simulink model "Dqo_model_Group_05"  (R2023a)
settings: Solver=VariableStepAuto  StartTime=0.0  StopTime=10.0  RelTol=1e-3
InitFcn:
  | Rs=0.03957
  | Rr=0.02215
  | Ls=0.000389+0.01664 %Lls+Lm
  | Lm=0.01664
  | Lr=0.000389+0.01664 % Llr+Lm
  | J=1.3
  | P=4
  | w=2*pi*60
  | Tl=200.106
settings Model: Creator=shivam  LastModifiedBy=shivam

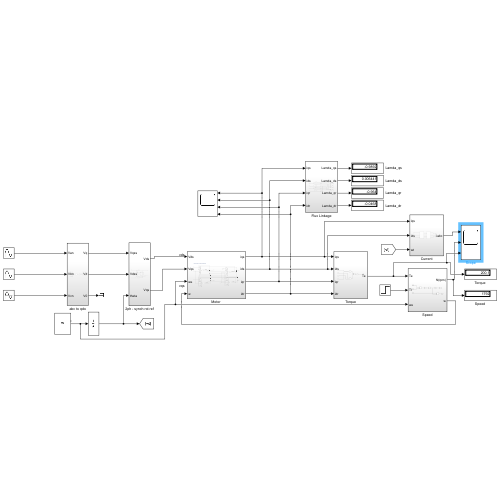
[thumbnail: Simulink's stored preview of the top-level diagram]
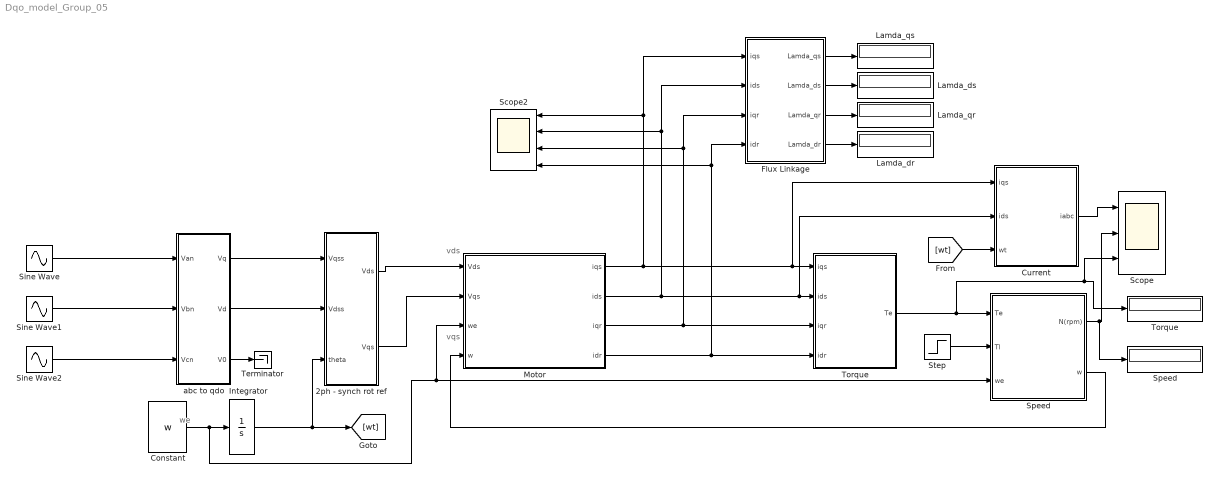
== system Dqo_model_Group_05 ==
  note: we
  note: vqs
  note: vds
  2ph - synch rot ref : Subsystem
  Constant : Constant  Value=w
  Current : Subsystem
  Flux Linkage : Subsystem
  Integrator : Integrator
  Lamda_dr : Display
  Lamda_ds : Display
  Lamda_qr : Display
  Lamda_qs : Display
  "Motor " : Subsystem
  Scope : Scope  NumInputPorts=3
  Scope2 : Scope  NumInputPorts=4
  Sine Wave : Sin  Amplitude=(460*sqrt(2))/sqrt(3)  Frequency=2*pi*60  SampleTime=0
  Sine Wave1 : Sin  Amplitude=(460*sqrt(2))/sqrt(3)  Frequency=2*pi*60  Phase=-(2*pi)/3  SampleTime=0
  Sine Wave2 : Sin  Amplitude=(460*sqrt(2))/sqrt(3)  Frequency=2*pi*60  Phase=(2*pi)/3  SampleTime=0
  Speed : Subsystem
  "Speed " : Display
  Step : Step  After=200.106  SampleTime=0
  Terminator : Terminator
  Torque : Subsystem
  "Torque " : Display
  abc to qdo : Subsystem
  wires:
  "Motor "/3(iqr) -> Torque/3(iqr), Scope2/3, Flux Linkage/3(iqr)
  abc to qdo/3(V0) -> Terminator/1
  2ph - synch rot ref/1(Vds) -> "Motor "/1("Vds ")
  Flux Linkage/4(Lamda_dr) -> Lamda_dr/1
  Speed/1(N(rpm)) -> "Speed "/1, Scope/2
  Constant/1 -> Speed/3(we), "Motor "/3(we), Integrator/1
  abc to qdo/1(Vq) -> 2ph - synch rot ref/1(Vqss)
  Speed/2(w) -> "Motor "/4(w)
  Torque/1("Te ") -> "Torque "/1, Scope/3, Speed/1(Te)
  Integrator/1 -> [wt], 2ph - synch rot ref/3(theta)
  Flux Linkage/1(Lamda_qs) -> Lamda_qs/1
  [wt] -> Current/3(wt)
  Step/1 -> Speed/2(Tl)
  Flux Linkage/2(Lamda_ds) -> Lamda_ds/1
  Sine Wave2/1 -> abc to qdo/3(Vcn)
  Sine Wave1/1 -> abc to qdo/2(Vbn)
  Current/1(iabc) -> Scope/1
  Flux Linkage/3(Lamda_qr) -> Lamda_qr/1
  "Motor "/4(idr) -> Torque/4(idr), Scope2/4, Flux Linkage/4(idr)
  2ph - synch rot ref/2(Vqs) -> "Motor "/2("Vqs ")
  Sine Wave/1 -> abc to qdo/1(Van)
  abc to qdo/2(Vd) -> 2ph - synch rot ref/2(Vdss)
  "Motor "/1(iqs) -> Current/1(iqs), Torque/1(iqs), Flux Linkage/1(iqs), Scope2/1
  "Motor "/2(ids) -> Current/2(ids), Torque/2(ids), Scope2/2, Flux Linkage/2(ids)

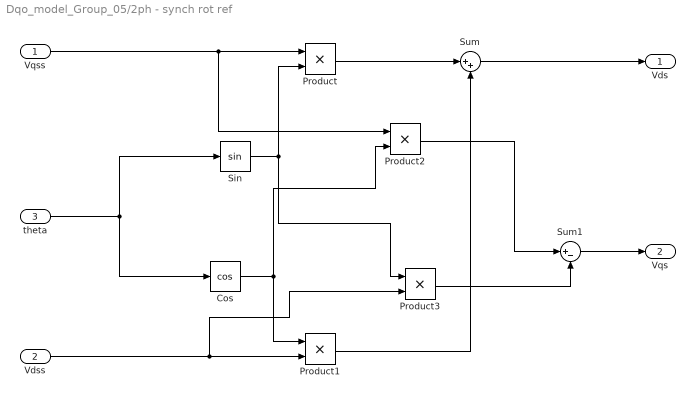
== system Dqo_model_Group_05/2ph - synch rot ref ==
  Vqss : Inport
  Vdss : Inport  Port=2
  theta : Inport  Port=3
  Cos : Trigonometry  Operator=cos
  Product{,1..3} (4 alike) : Product
  Sin : Trigonometry
  Sum : Sum  Inputs=|++
  Sum1 : Sum  Inputs=|+-
  Vds : Outport
  Vqs : Outport  Port=2
  wires:
  theta/1 -> Sin/1, Cos/1
  Vqss/1 -> Product2/1, Product/1
  Sin/1 -> Product/2, Product3/1
  Vdss/1 -> Product3/2, Product1/2
  Cos/1 -> Product1/1, Product2/2
  Product/1 -> Sum/1
  Product1/1 -> Sum/2
  Sum/1 -> Vds/1
  Product2/1 -> Sum1/1
  Product3/1 -> Sum1/2
  Sum1/1 -> Vqs/1

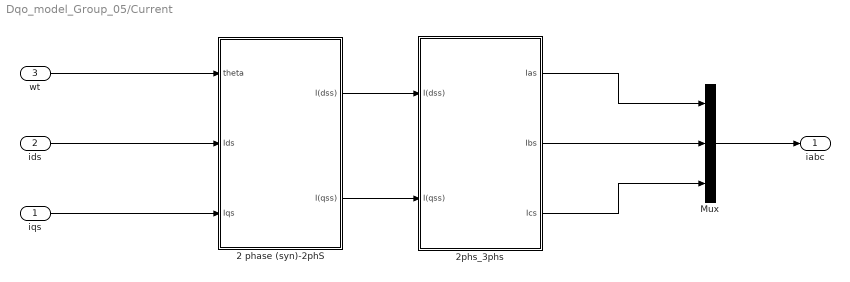
== system Dqo_model_Group_05/Current ==
  iqs : Inport
  ids : Inport  Port=2
  wt : Inport  Port=3
  2 phase (syn)-2phS : Subsystem
  2phs_3phs : Subsystem
  Mux : Mux  Inputs=3
  iabc : Outport  VectorParamsAs1DForOutWhenUnconnected=off
  wires:
  ids/1 -> 2 phase (syn)-2phS/2(Ids)
  iqs/1 -> 2 phase (syn)-2phS/3(Iqs)
  wt/1 -> 2 phase (syn)-2phS/1(theta)
  Mux/1 -> iabc/1
  2 phase (syn)-2phS/1(I(dss)) -> 2phs_3phs/1(I(dss))
  2 phase (syn)-2phS/2(I(qss)) -> 2phs_3phs/2(I(qss))
  2phs_3phs/1(Ias) -> Mux/1
  2phs_3phs/2(Ibs) -> Mux/2
  2phs_3phs/3(Ics) -> Mux/3

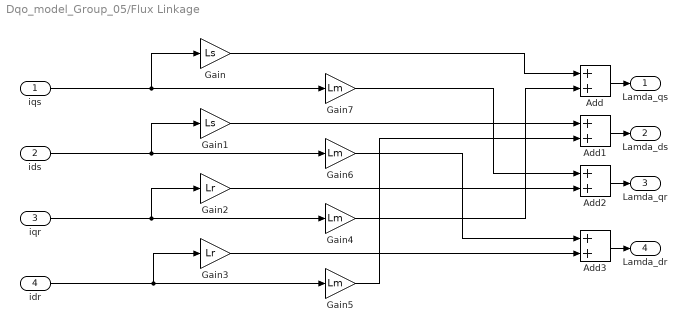
== system Dqo_model_Group_05/Flux Linkage ==
  iqs : Inport
  ids : Inport  Port=2
  iqr : Inport  Port=3
  idr : Inport  Port=4
  Add{,1..3} (4 alike) : Sum
  Gain : Gain  Gain=Ls
  Gain1 : Gain  Gain=Ls
  Gain2 : Gain  Gain=Lr
  Gain3 : Gain  Gain=Lr
  Gain{4..7} (4 alike) : Gain  Gain=Lm
  Lamda_qs : Outport
  Lamda_ds : Outport  Port=2
  Lamda_qr : Outport  Port=3
  Lamda_dr : Outport  Port=4
  wires:
  Gain4/1 -> Add/2
  Gain1/1 -> Add1/1
  ids/1 -> Gain6/1, Gain1/1
  iqs/1 -> Gain7/1, Gain/1
  Gain6/1 -> Add3/1
  idr/1 -> Gain5/1, Gain3/1
  iqr/1 -> Gain4/1, Gain2/1
  Gain5/1 -> Add1/2
  Gain/1 -> Add/1
  Gain7/1 -> Add2/1
  Gain3/1 -> Add3/2
  Add2/1 -> Lamda_qr/1
  Gain2/1 -> Add2/2
  Add/1 -> Lamda_qs/1
  Add3/1 -> Lamda_dr/1
  Add1/1 -> Lamda_ds/1

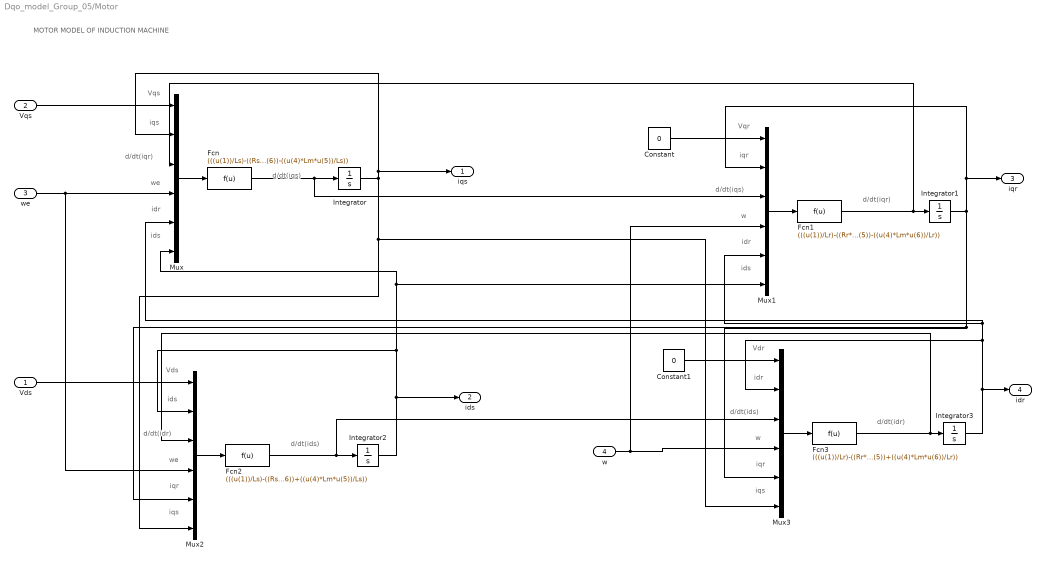
== system Dqo_model_Group_05/Motor  ==
  note: d/dt(iqs)
  note: ids
  note: idr
  note: we
  note: d/dt(iqr)
  note: iqs
  note: Vqs
  note: MOTOR MODEL OF INDUCTION MACHINE
  note: d/dt(iqr)
  note: ids
  note: d/dt(iqs)
  note: w
  note: idr
  note: Vqr
  note: iqr
  note: d/dt(ids)
  note: iqs
  note: d/dt(idr)
  note: we
  note: iqr
  note: Vds
  note: ids
  note: iqr
  note: w
  note: Vdr
  note: d/dt(ids)
  note: idr
  note: iqs
  note: d/dt(idr)
  "Vds " : Inport
  "Vqs " : Inport  Port=2
  we : Inport  Port=3
  w : Inport  Port=4
  Constant : Constant  Value=0
  Constant1 : Constant  Value=0
  Fcn : Fcn  Expr=(((u(1))/Ls)-((Rs*u(2))/Ls)-((u(3)*Lm)/Ls)-(u(4)*u(6))-((u(4)*Lm*u(5))/Ls))
  Fcn1 : Fcn  Expr=(((u(1))/Lr)-((Rr*u(2))/Lr)-((u(3)*Lm)/Lr)-(u(4)*u(5))-((u(4)*Lm*u(6))/Lr))
  Fcn2 : Fcn  Expr=(((u(1))/Ls)-((Rs*u(2))/Ls)-((u(3)*Lm)/Ls)+(u(4)*u(6))+((u(4)*Lm*u(5))/Ls))
  Fcn3 : Fcn  Expr=(((u(1))/Lr)-((Rr*u(2))/Lr)-((u(3)*Lm)/Lr)+(u(4)*u(5))+((u(4)*Lm*u(6))/Lr))
  Integrator{,1..3} (4 alike) : Integrator
  Mux{,1..3} (4 alike) : Mux  Inputs=6
  iqs : Outport  VectorParamsAs1DForOutWhenUnconnected=off
  ids : Outport  Port=2  VectorParamsAs1DForOutWhenUnconnected=off
  iqr : Outport  Port=3  VectorParamsAs1DForOutWhenUnconnected=off
  idr : Outport  Port=4  VectorParamsAs1DForOutWhenUnconnected=off
  wires:
  Integrator3/1 -> idr/1, Mux3/2, Mux1/5, Mux/5
  Mux/1 -> Fcn/1
  Fcn2/1 -> Mux3/3, Integrator2/1
  Integrator/1 -> iqs/1, Mux/2, Mux3/6, Mux2/6
  Integrator2/1 -> ids/1, Mux1/6, Mux/6, Mux2/2
  Integrator1/1 -> iqr/1, Mux1/2, Mux3/5, Mux2/5
  Constant/1 -> Mux1/1
  w/1 -> Mux1/4, Mux3/4
  "Vds "/1 -> Mux2/1
  Fcn3/1 -> Mux2/3, Integrator3/1
  Constant1/1 -> Mux3/1
  Fcn1/1 -> Mux/3, Integrator1/1
  "Vqs "/1 -> Mux/1
  Mux2/1 -> Fcn2/1
  Mux3/1 -> Fcn3/1
  we/1 -> Mux2/4, Mux/4
  Fcn/1 -> Mux1/3, Integrator/1
  Mux1/1 -> Fcn1/1

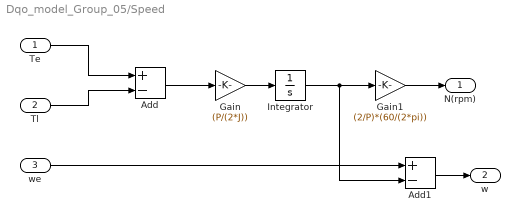
== system Dqo_model_Group_05/Speed ==
  Te : Inport
  Tl : Inport  Port=2
  we : Inport  Port=3
  Add : Sum  Inputs=+-
  Add1 : Sum  Inputs=+-
  Gain : Gain  Gain=(P/(2*J))
  Gain1 : Gain  Gain=(2/P)*(60/(2*pi))
  Integrator : Integrator
  N(rpm) : Outport  VectorParamsAs1DForOutWhenUnconnected=off
  w : Outport  Port=2  VectorParamsAs1DForOutWhenUnconnected=off
  wires:
  we/1 -> Add1/1
  Tl/1 -> Add/2
  Integrator/1 -> Add1/2, Gain1/1
  Te/1 -> Add/1
  Add/1 -> Gain/1
  Gain1/1 -> N(rpm)/1
  Gain/1 -> Integrator/1
  Add1/1 -> w/1

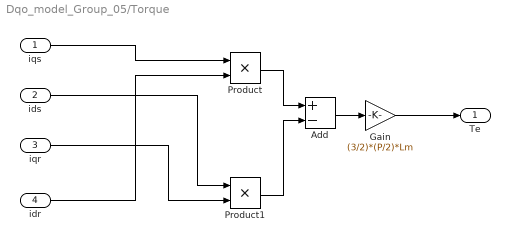
== system Dqo_model_Group_05/Torque ==
  iqs : Inport
  ids : Inport  Port=2
  iqr : Inport  Port=3
  idr : Inport  Port=4
  Add : Sum  Inputs=+-
  Gain : Gain  Gain=(3/2)*(P/2)*Lm
  Product : Product
  Product1 : Product
  "Te " : Outport  VectorParamsAs1DForOutWhenUnconnected=off
  wires:
  ids/1 -> Product1/1
  Product1/1 -> Add/2
  iqr/1 -> Product1/2
  idr/1 -> Product/2
  iqs/1 -> Product/1
  Gain/1 -> "Te "/1
  Add/1 -> Gain/1
  Product/1 -> Add/1

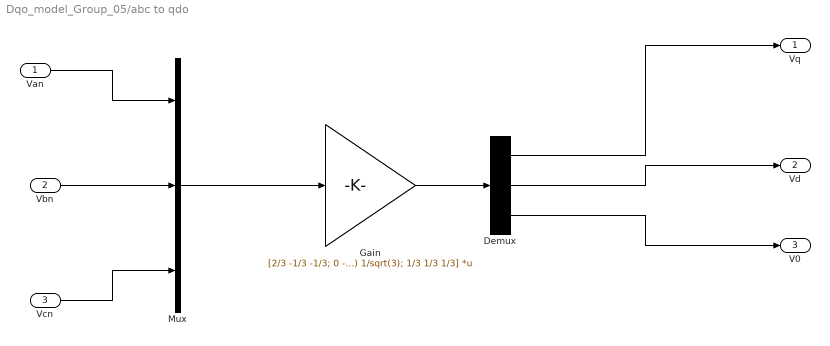
== system Dqo_model_Group_05/abc to qdo ==
  Van : Inport
  Vbn : Inport  Port=2
  Vcn : Inport  Port=3
  Demux : Demux  Outputs=3
  Gain : Gain  Gain=[2/3 -1/3 -1/3; 0 -1/sqrt(3) 1/sqrt(3); 1/3 1/3 1/3]  Multiplication=Matrix(K*u)
  Mux : Mux  Inputs=3
  Vq : Outport
  Vd : Outport  Port=2
  V0 : Outport  Port=3
  wires:
  Vbn/1 -> Mux/2
  Vcn/1 -> Mux/3
  Van/1 -> Mux/1
  Mux/1 -> Gain/1
  Gain/1 -> Demux/1
  Demux/1 -> Vq/1
  Demux/2 -> Vd/1
  Demux/3 -> V0/1

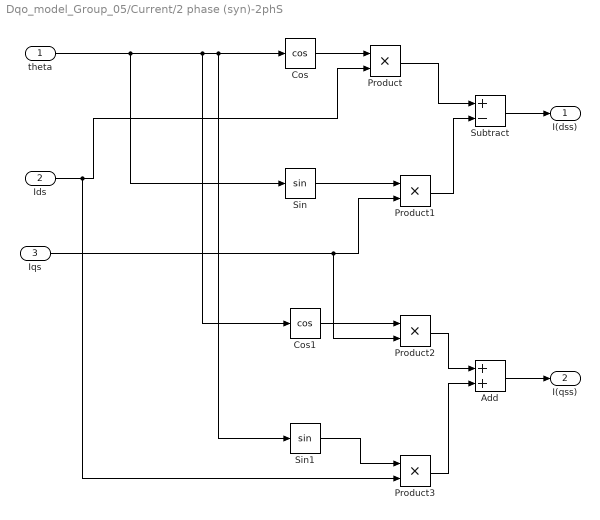
== system Dqo_model_Group_05/Current/2 phase (syn)-2phS ==
  theta : Inport
  Ids : Inport  Port=2
  Iqs : Inport  Port=3
  Add : Sum
  Cos : Trigonometry  Operator=cos
  Cos1 : Trigonometry  Operator=cos
  Product{,1..3} (4 alike) : Product
  Sin : Trigonometry
  Sin1 : Trigonometry
  Subtract : Sum  Inputs=+-
  I(dss) : Outport
  I(qss) : Outport  Port=2
  wires:
  theta/1 -> Sin/1, Cos1/1, Sin1/1, Cos/1
  Sin/1 -> Product1/1
  Iqs/1 -> Product2/2, Product1/2
  Cos/1 -> Product/1
  Ids/1 -> Product3/2, Product/2
  Product/1 -> Subtract/1
  Product1/1 -> Subtract/2
  Subtract/1 -> I(dss)/1
  Cos1/1 -> Product2/1
  Sin1/1 -> Product3/1
  Product2/1 -> Add/1
  Product3/1 -> Add/2
  Add/1 -> I(qss)/1

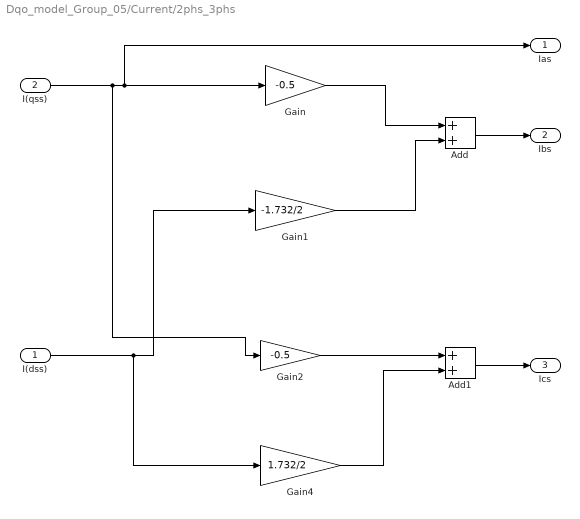
== system Dqo_model_Group_05/Current/2phs_3phs ==
  I(dss) : Inport
  I(qss) : Inport  Port=2
  Add : Sum
  Add1 : Sum
  Gain : Gain  Gain=-0.5
  Gain1 : Gain  Gain=-1.732/2
  Gain2 : Gain  Gain=-0.5
  Gain4 : Gain  Gain=1.732/2
  Ias : Outport
  Ibs : Outport  Port=2
  Ics : Outport  Port=3
  wires:
  I(qss)/1 -> Ias/1, Gain/1, Gain2/1
  I(dss)/1 -> Gain4/1, Gain1/1
  Gain/1 -> Add/1
  Gain1/1 -> Add/2
  Gain2/1 -> Add1/1
  Gain4/1 -> Add1/2
  Add/1 -> Ibs/1
  Add1/1 -> Ics/1
